simulink model "SS_angulo_pos_planta_OPENLOOP_simulink"  (R2023b)
settings: Solver=VariableStepAuto  StartTime=0.0  StopTime=15  RelTol=1e-6
values from neighbouring files (symbols this model uses):
  Planta = ss([0 0 1 0;0 0 0 1;0 0 -11.48 0;0 -35.39 0 -0.01639],[0;-0.3736;0.2846;-0.8948],[1 0 0 0;0 1 0 0],0)    [Script_generador.m]
undefined symbols (not defined in the file or in its folder): SS_An, SS_Po
settings Model: Creator=natih  LastModifiedBy=jmarin

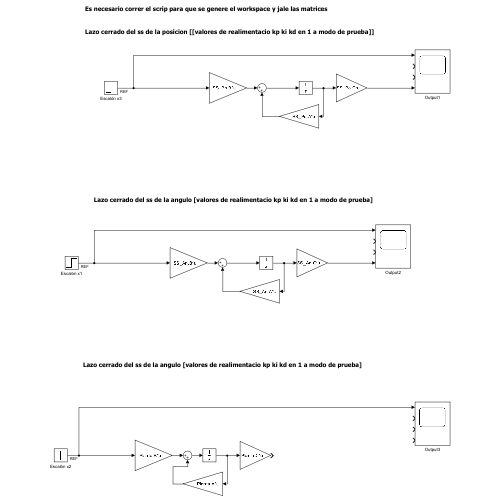
[thumbnail: Simulink's stored preview of the top-level diagram]
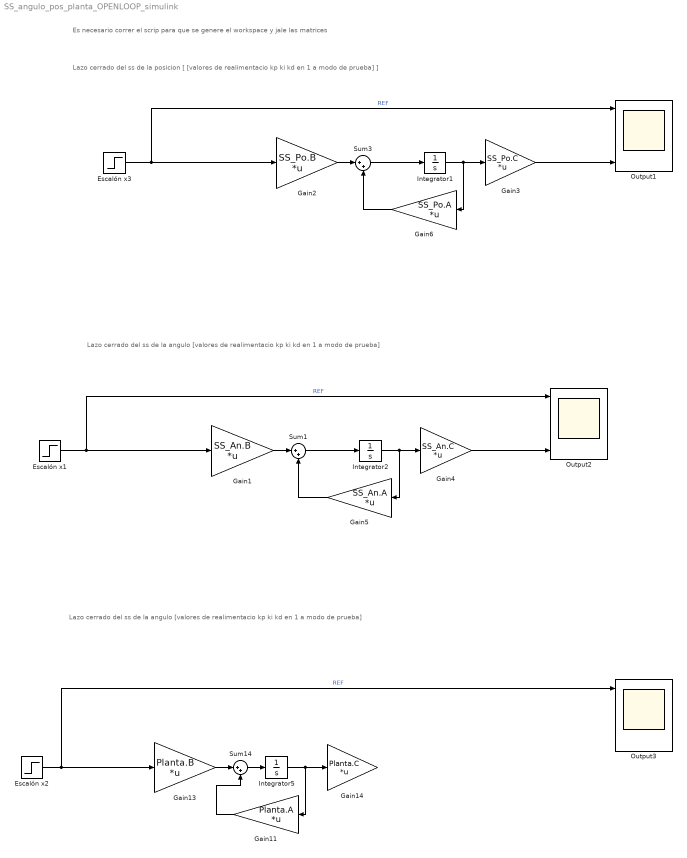
== system SS_angulo_pos_planta_OPENLOOP_simulink ==
  note: Lazo cerrado del ss de la posicion [ [valores de realimentacio kp ki kd en 1 a modo de prueba] ]
  note: Lazo cerrado del ss de la angulo [valores de realimentacio kp ki kd en 1 a modo de prueba]
  note: Es necesario correr el scrip para que se genere el workspace y jale las matrices
  note: Lazo cerrado del ss de la angulo [valores de realimentacio kp ki kd en 1 a modo de prueba]
  Escalón x1 : Step  Time=0.5  SampleTime=0
  Escalón x2 : Step  Time=0.5  SampleTime=0
  Escalón x3 : Step  Time=0.5  SampleTime=0
  Gain1 : Gain  Gain=SS_An.B  Multiplication=Matrix(K*u)
  Gain11 : Gain  Gain=Planta.A  Multiplication=Matrix(K*u)
  Gain13 : Gain  Gain=Planta.B  Multiplication=Matrix(K*u)
  Gain14 : Gain  Gain=Planta.C  Multiplication=Matrix(K*u)
  Gain2 : Gain  Gain=SS_Po.B  Multiplication=Matrix(K*u)
  Gain3 : Gain  Gain=SS_Po.C  Multiplication=Matrix(K*u)
  Gain4 : Gain  Gain=SS_An.C  Multiplication=Matrix(K*u)
  Gain5 : Gain  Gain=SS_An.A  Multiplication=Matrix(K*u)
  Gain6 : Gain  Gain=SS_Po.A  Multiplication=Matrix(K*u)
  Integrator1 : Integrator
  Integrator2 : Integrator
  Integrator5 : Integrator
  Output1 : Scope  NumInputPorts=4
  Output2 : Scope  NumInputPorts=4
  Output3 : Scope  NumInputPorts=4
  Sum1 : Sum  Inputs=|++
  Sum14 : Sum  Inputs=|++
  Sum3 : Sum  Inputs=|++
  wires:
  Escalón x3/1 -> Output1/1, Gain2/1  "REF"
  Gain2/1 -> Sum3/1
  Sum3/1 -> Integrator1/1
  Integrator1/1 -> Gain6/1, Gain3/1
  Gain3/1 -> Output1/4
  Gain6/1 -> Sum3/2
  Escalón x2/1 -> Gain13/1, Output3/1  "REF"
  Integrator5/1 -> Gain11/1, Gain14/1
  Gain13/1 -> Sum14/1
  Sum14/1 -> Integrator5/1
  Gain11/1 -> Sum14/2
  Integrator2/1 -> Gain5/1, Gain4/1
  Sum1/1 -> Integrator2/1
  Gain5/1 -> Sum1/2
  Escalón x1/1 -> Output2/1, Gain1/1  "REF"
  Gain4/1 -> Output2/4
  Gain1/1 -> Sum1/1
